simulink model "kr_billiards_debug"  (R2017b)
settings: Solver=VariableStepAuto  StartTime=0.0  StopTime=40  RelTol=1e-3  EnableMultiTasking=on
PreLoadFcn:
  | addpath('Bill_Tables_STEP')
  | addpath('Skins')
  | addpath('Utilities')
  | addpath('Kuka_KR10_R1100_STEP')
model workspace (MATLAB code in the model file):
  | den=1.613292710828678e+03;
  | st=0.004;
  | Damping=0.2;
  | 
  | % Length of brick solid
  | L = 20; % cm
  | % Width of brick solid
  | W = 2; % cm
  | % Height of brick solid
  | H = 2; % cm
  | % Density of brick solid
  | rho = 1000; % kg/m^3
undefined symbols (not defined in the file or in its folder): ball_col, ball_x, ball_y, X, Y, Z
libraries: sm_lib x83, nesl_utility x64, fl_lib x12, simulink x4
(part 4 of 4)

== matlab function kr_billiards_debug/Billiards/MATLAB Function1 ==
  data: x0 input; y0 input; z0 input; x input; Fx output; y input; Fy output; U output
function [Fx, Fy, U] = fcn(x0, y0, z0, x, y)

R=0.034;  % радиус шара
%k=5000;
k=10000; % коэффициент упругости шар-шар
kb=10000; % коэффициент упругости борт-шар
kp=100; % коэффициент притяжения в центр лузы

RL=[0.1 0.1 0.065 0.1 0.1 0.065].^2;  % радиус луз в квадрате (из-за углубления угловые лузы "больше")


x_min=0.333;
x_max=1.116;
y_min=-0.8065;
y_max=0.8065;



s=0.051; % смещение лузы от борта 

% центры луз
Lx=[x_min-s x_max+s x_max+s x_max+s x_min-s x_min-s];
Ly=[y_max+s y_max+s 0 y_min-s y_min-s 0];


n=length(x);
Fx=zeros(n,1);
Fy=zeros(n,1);
z=0.103;  % 0.103 - уровень шаров по координате z 


U=zeros(n,1);  % 1 если шар в лузе

% попадания в лузы
for i=1:n
    for j=1:6
        dx=Lx(j)-x(i);
        dy=Ly(j)-y(i);
        if dx^2+dy^2<RL(j)
            U(i)=1;
            Fx(i)=dx*kp;
            Fy(i)=dy*kp;
        end
    end
    if U(i)==0 % если шар не в лузе, то проверяем удары об борта (упругий удар)
        Fx(i)=Fx(i)+kb*(x_min-x(i))*((x_min-x(i))>0)-kb*(x(i)-x_max)*((x(i)-x_max)>0);
        Fy(i)=Fy(i)+kb*(y_min-y(i))*((y_min-y(i))>0)-kb*(y(i)-y_max)*((y(i)-y_max)>0);       
    end
end


% биток по шарам
for i=1:n
    if U(i)==0
        dx=x0-x(i);
        dy=y0-y(i);
        r=sqrt(dx^2+dy^2+(z-z0)^2);
        d=r-2*R;
        if d<0
            Fx(i)=Fx(i)+k*d*dx/r;
            Fy(i)=Fy(i)+k*d*dy/r;
        end
    end
end



% соударения
for i=1:n-1
    if U(i)==0
        for j=i+1:n
            if U(j)==0
                dx=x(i)-x(j);
                dy=y(i)-y(j);
                r=sqrt(dx^2+dy^2);
                d=r-2*R;
                if d<0
                    fx=k*d*dx/r;
                    fy=k*d*dy/r;
                    Fx(i)=Fx(i)-fx;
                    Fx(j)=Fx(j)+fx;
                    Fy(i)=Fy(i)-fy;
                    Fy(j)=Fy(j)+fy;
                end
            end
        end
    end
end
